simulink model "radar_distributed"  (R2025b)
settings: Solver=FixedStepDiscrete  StartTime=0.0  StopTime=16  FixedStep=0.04  RelTol=1e-3
InitFcn:
  | addpath('C:\Users\Meric\Documents\GitHub\Radar-Distributed-Architecture\simulink'); radar_sim_reset;
settings Model: Creator=Meric  LastModifiedBy=Meric

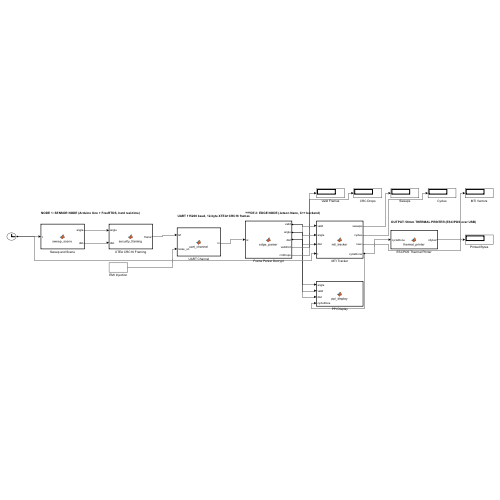
[thumbnail: Simulink's stored preview of the top-level diagram]
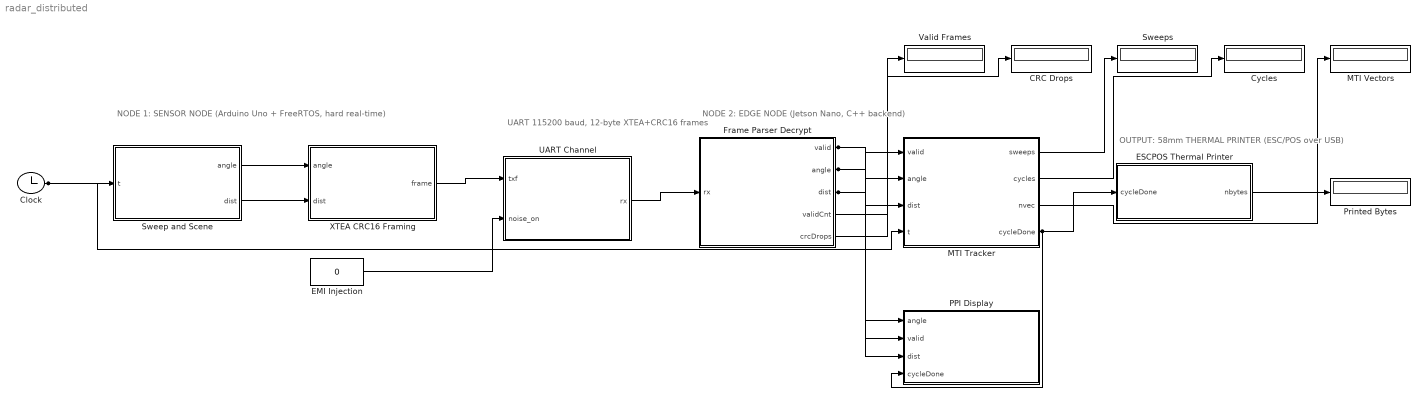
== system radar_distributed ==
  note: NODE 1: SENSOR NODE (Arduino Uno + FreeRTOS, hard real-time)
  note: UART 115200 baud, 12-byte XTEA+CRC16 frames
  note: NODE 2: EDGE NODE (Jetson Nano, C++ backend)
  note: OUTPUT: 58mm THERMAL PRINTER (ESC/POS over USB)
  CRC Drops : Display
  Clock : Clock
  Cycles : Display
  EMI Injection : Constant  Value=0
  ESCPOS Thermal Printer : MATLAB Function  TreatAsAtomicUnit=on
  Frame Parser Decrypt : MATLAB Function  TreatAsAtomicUnit=on
  MTI Tracker : MATLAB Function  TreatAsAtomicUnit=on
  MTI Vectors : Display
  PPI Display : MATLAB Function  TreatAsAtomicUnit=on
  Printed Bytes : Display
  Sweep and Scene : MATLAB Function  TreatAsAtomicUnit=on
  Sweeps : Display
  UART Channel : MATLAB Function  TreatAsAtomicUnit=on
  Valid Frames : Display
  XTEA CRC16 Framing : MATLAB Function  TreatAsAtomicUnit=on
  wires:
  Clock/1 -> Sweep and Scene/1(t), MTI Tracker/4(t)
  Sweep and Scene/1(angle) -> XTEA CRC16 Framing/1(angle)
  Sweep and Scene/2(dist) -> XTEA CRC16 Framing/2(dist)
  XTEA CRC16 Framing/1(frame) -> UART Channel/1(txf)
  EMI Injection/1 -> UART Channel/2(noise_on)
  UART Channel/1(rx) -> Frame Parser Decrypt/1(rx)
  Frame Parser Decrypt/1(valid) -> MTI Tracker/1(valid), PPI Display/2(valid)
  Frame Parser Decrypt/2(angle) -> MTI Tracker/2(angle), PPI Display/1(angle)
  Frame Parser Decrypt/3(dist) -> MTI Tracker/3(dist), PPI Display/3(dist)
  Frame Parser Decrypt/4(validCnt) -> Valid Frames/1
  Frame Parser Decrypt/5(crcDrops) -> CRC Drops/1
  MTI Tracker/1(sweeps) -> Sweeps/1
  MTI Tracker/2(cycles) -> Cycles/1
  MTI Tracker/3(nvec) -> MTI Vectors/1
  MTI Tracker/4(cycleDone) -> PPI Display/4(cycleDone), ESCPOS Thermal Printer/1(cycleDone)
  ESCPOS Thermal Printer/1(nbytes) -> Printed Bytes/1

== matlab function radar_distributed/XTEA CRC16 Framing ==
  data: angle input; frame output; dist input
function frame = security_framing(angle, dist)
% TaskSecurity equivalent: XTEA-encrypted 12-byte telemetry frame.
coder.extrinsic('radar_build_frame');
frame = zeros(12, 1);
frame = radar_build_frame(angle, dist);
end

== matlab function radar_distributed/Sweep and Scene ==
  data: t input; angle output; dist output
function [angle, dist] = sweep_scene(t)
% Servo triangle sweep, 2 deg per 40 ms step (sketch_may7d timing),
% plus the simulated HC-SR04 echo from the tabletop target scene.
coder.extrinsic('radar_scene');
step = floor(t / 0.04);
phase = mod(step * 2, 360);
if phase <= 180
    angle = phase;
else
    angle = 360 - phase;
end
dist = 0;
dist = radar_scene(angle, t);
end

== matlab function radar_distributed/UART Channel ==
  data: txf input; rx output; noise_on input
function rx = uart_channel(txf, noise_on)
% 115200-baud link; EMI Injection = 1 flips random bits (Metric 1).
coder.extrinsic('radar_channel');
rx = zeros(12, 1);
rx = radar_channel(txf, noise_on);
end

== matlab function radar_distributed/Frame Parser Decrypt ==
  data: rx input; valid output; angle output; dist output; validCnt output; crcDrops output
function [valid, angle, dist, validCnt, crcDrops] = edge_parser(rx)
% Backend FrameParser equivalent: sync + CRC check, XTEA decrypt.
coder.extrinsic('radar_parse_frame');
valid = 0; angle = 0; dist = 0; validCnt = 0; crcDrops = 0;
[valid, angle, dist, validCnt, crcDrops] = radar_parse_frame(rx);
end

== matlab function radar_distributed/MTI Tracker ==
  data: valid input; sweeps output; angle input; dist input; t input; cycles output; nvec output; cycleDone output
function [sweeps, cycles, nvec, cycleDone] = mti_tracker(valid, angle, dist, t)
% SweepBuilder + nearest-neighbor MTI (backend mti_cpu equivalent).
coder.extrinsic('radar_mti_step');
sweeps = 0; cycles = 0; nvec = 0; cycleDone = 0;
[sweeps, cycles, nvec, cycleDone] = radar_mti_step(valid, angle, dist, t);
end

== matlab function radar_distributed/PPI Display ==
  data: angle input; valid input; dist input; cycleDone input
function ppi_display(angle, valid, dist, cycleDone)
% Live half-PPI preview (stand-in for the Vulkan renderer).
coder.extrinsic('radar_ppi_draw');
radar_ppi_draw(angle, valid, dist, cycleDone);
end

== matlab function radar_distributed/ESCPOS Thermal Printer ==
  data: cycleDone input; nbytes output
function nbytes = thermal_printer(cycleDone)
% Stage 5: on each completed bidirectional cycle, rasterize the PPI,
% encode real ESC/POS bytes, and send them to the virtual printer.
coder.extrinsic('radar_escpos_encode', 'radar_virtual_printer');
nbytes = 0;
if cycleDone > 0.5
    b = radar_escpos_encode();
    nbytes = radar_virtual_printer(b);
end
end
